simulink model "Continuous_sim"  (R2025a)
settings: Solver=VariableStepAuto  StartTime=0.0  StopTime=20  RelTol=1e-3
settings Model: Creator=user  LastModifiedBy=user

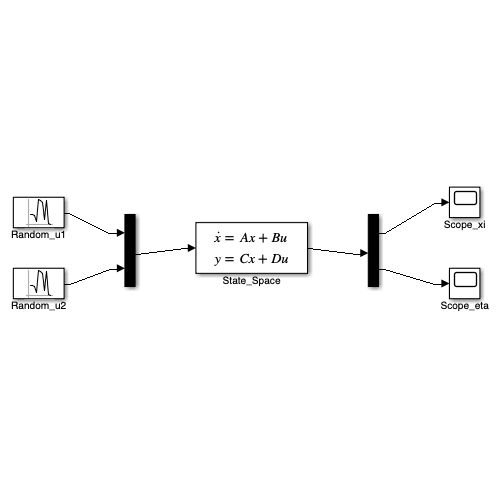
[thumbnail: Simulink's stored preview of the top-level diagram]
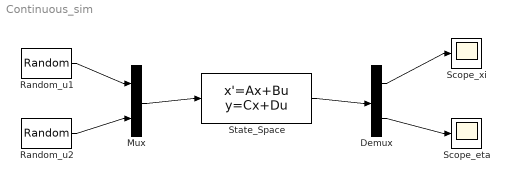
== system Continuous_sim ==
  Demux : Demux  Outputs=2
  Mux : Mux  Inputs=2
  Random_u1 : RandomNumber  SampleTime=0.1
  Random_u2 : RandomNumber  SampleTime=0.1
  Scope_eta : Scope
  Scope_xi : Scope
  State_Space : StateSpace  A=[0 1 0 0;0 0 0 -0.5;0 0 0 1;0 0.5 0 0]  B=[0 0;1 0;0 0;0 1]  C=[1 0 0 0;0 0 1 0]  D=[0 0;0 0]  InitialCondition=[0 0.1 0 0.1]
  wires:
  Random_u1/1 -> Mux/1
  Random_u2/1 -> Mux/2
  Mux/1 -> State_Space/1
  State_Space/1 -> Demux/1
  Demux/1 -> Scope_xi/1
  Demux/2 -> Scope_eta/1
